simulink model "TotalAssemblyV4"  (R2020b)
settings: Solver=VariableStepAuto  StartTime=0.0  StopTime=10.0  RelTol=1e-3
model workspace: external: MATLAB File C:\Users\User\Aalborg Universitet\ROB 3 - General\P3\Solidworks_files\SimScapeV4\TotalAssemblyV4_DataFile.m (data not in the file)
undefined symbols (not defined in the file or in its folder): smiData, X, Y, Z
libraries: sm_lib x112, simulink_extras x16, nesl_utility x13
(part 3 of 3)

== system TotalAssemblyV4/Body3_3_RIGID/Servo_Disc_3_RIGID ==
  ReferenceFrame : sm_lib/Frames and Transforms/Reference Frame
  Solid : sm_lib/Body Elements/File Solid  ExtGeomFileName=Servo-Disc_Default_sldprt.STEP  UnitType=FromFile  ExtGeomFileUnits=m  StepReaderType=HEX  ExportConvexHullGeometry=off  InertiaType=Custom  Mass=smiData.Solid(2).mass  MassUnits=kg  CenterOfMass=smiData.Solid(2).CoM  CenterOfMassUnits=mm  MomentsOfInertia=smiData.Solid(2).MoI  MomentsOfInertiaUnits=kg*mm^2  ProductsOfInertia=smiData.Solid(2).PoI  ProductsOfInertiaUnits=kg*mm^2  BasedOnType=DensityFromFile  Density=1000  DensityUnits=kg/m^3  DoExposeReferenceFrame=on  SerializedFrames=<Frames/>  GraphicType=FromGeometry  MarkerShape=Sphere  MarkerSize=10  GraphicVisPropType=SimpleVisualProperties  GraphicDiffuseColor=smiData.Solid(2).color  GraphicSpecularColor=[0.5 0.5 0.5 1.0]  GraphicAmbientColor=[0.15 0.15 0.15 1.0]  GraphicEmissiveColor=[0.0 0.0 0.0 1.0]  GraphicShininess=75  GraphicOpacity=smiData.Solid(2).opacity
  F : PMIOPort  Side=Left
  connections:
  Solid/RConn1 -- ReferenceFrame/RConn1 -- F/RConn1

== system TotalAssemblyV4/Body3_3_RIGID/Servo_Disc_4_RIGID ==
  ReferenceFrame : sm_lib/Frames and Transforms/Reference Frame
  Solid : sm_lib/Body Elements/File Solid  ExtGeomFileName=Servo-Disc_Default_sldprt.STEP  UnitType=FromFile  ExtGeomFileUnits=m  StepReaderType=HEX  ExportConvexHullGeometry=off  InertiaType=Custom  Mass=smiData.Solid(2).mass  MassUnits=kg  CenterOfMass=smiData.Solid(2).CoM  CenterOfMassUnits=mm  MomentsOfInertia=smiData.Solid(2).MoI  MomentsOfInertiaUnits=kg*mm^2  ProductsOfInertia=smiData.Solid(2).PoI  ProductsOfInertiaUnits=kg*mm^2  BasedOnType=DensityFromFile  Density=1000  DensityUnits=kg/m^3  DoExposeReferenceFrame=on  SerializedFrames=<Frames/>  GraphicType=FromGeometry  MarkerShape=Sphere  MarkerSize=10  GraphicVisPropType=SimpleVisualProperties  GraphicDiffuseColor=smiData.Solid(2).color  GraphicSpecularColor=[0.5 0.5 0.5 1.0]  GraphicAmbientColor=[0.15 0.15 0.15 1.0]  GraphicEmissiveColor=[0.0 0.0 0.0 1.0]  GraphicShininess=75  GraphicOpacity=smiData.Solid(2).opacity
  F : PMIOPort  Side=Left
  connections:
  Solid/RConn1 -- ReferenceFrame/RConn1 -- F/RConn1

== system TotalAssemblyV4/Body3_3_RIGID/Servo_Disc_5_RIGID ==
  ReferenceFrame : sm_lib/Frames and Transforms/Reference Frame
  Solid : sm_lib/Body Elements/File Solid  ExtGeomFileName=Servo-Disc_Default_sldprt.STEP  UnitType=FromFile  ExtGeomFileUnits=m  StepReaderType=HEX  ExportConvexHullGeometry=off  InertiaType=Custom  Mass=smiData.Solid(2).mass  MassUnits=kg  CenterOfMass=smiData.Solid(2).CoM  CenterOfMassUnits=mm  MomentsOfInertia=smiData.Solid(2).MoI  MomentsOfInertiaUnits=kg*mm^2  ProductsOfInertia=smiData.Solid(2).PoI  ProductsOfInertiaUnits=kg*mm^2  BasedOnType=DensityFromFile  Density=1000  DensityUnits=kg/m^3  DoExposeReferenceFrame=on  SerializedFrames=<Frames/>  GraphicType=FromGeometry  MarkerShape=Sphere  MarkerSize=10  GraphicVisPropType=SimpleVisualProperties  GraphicDiffuseColor=smiData.Solid(2).color  GraphicSpecularColor=[0.5 0.5 0.5 1.0]  GraphicAmbientColor=[0.15 0.15 0.15 1.0]  GraphicEmissiveColor=[0.0 0.0 0.0 1.0]  GraphicShininess=75  GraphicOpacity=smiData.Solid(2).opacity
  F : PMIOPort  Side=Left
  connections:
  Solid/RConn1 -- ReferenceFrame/RConn1 -- F/RConn1

== system TotalAssemblyV4/Body3_3_RIGID/Servo_Disc_6_RIGID ==
  ReferenceFrame : sm_lib/Frames and Transforms/Reference Frame
  Solid : sm_lib/Body Elements/File Solid  ExtGeomFileName=Servo-Disc_Default_sldprt.STEP  UnitType=FromFile  ExtGeomFileUnits=m  StepReaderType=HEX  ExportConvexHullGeometry=off  InertiaType=Custom  Mass=smiData.Solid(2).mass  MassUnits=kg  CenterOfMass=smiData.Solid(2).CoM  CenterOfMassUnits=mm  MomentsOfInertia=smiData.Solid(2).MoI  MomentsOfInertiaUnits=kg*mm^2  ProductsOfInertia=smiData.Solid(2).PoI  ProductsOfInertiaUnits=kg*mm^2  BasedOnType=DensityFromFile  Density=1000  DensityUnits=kg/m^3  DoExposeReferenceFrame=on  SerializedFrames=<Frames/>  GraphicType=FromGeometry  MarkerShape=Sphere  MarkerSize=10  GraphicVisPropType=SimpleVisualProperties  GraphicDiffuseColor=smiData.Solid(2).color  GraphicSpecularColor=[0.5 0.5 0.5 1.0]  GraphicAmbientColor=[0.15 0.15 0.15 1.0]  GraphicEmissiveColor=[0.0 0.0 0.0 1.0]  GraphicShininess=75  GraphicOpacity=smiData.Solid(2).opacity
  F : PMIOPort  Side=Left
  connections:
  Solid/RConn1 -- ReferenceFrame/RConn1 -- F/RConn1

== system TotalAssemblyV4/Body3_3_RIGID/Servo_disc_link_MX_28T_1_RIGID ==
  ReferenceFrame : sm_lib/Frames and Transforms/Reference Frame
  Solid : sm_lib/Body Elements/File Solid  ExtGeomFileName=Servo-disc-link_MX-28T_Default_sldprt.STEP  UnitType=FromFile  ExtGeomFileUnits=m  StepReaderType=HEX  ExportConvexHullGeometry=off  InertiaType=Custom  Mass=smiData.Solid(15).mass  MassUnits=kg  CenterOfMass=smiData.Solid(15).CoM  CenterOfMassUnits=mm  MomentsOfInertia=smiData.Solid(15).MoI  MomentsOfInertiaUnits=kg*mm^2  ProductsOfInertia=smiData.Solid(15).PoI  ProductsOfInertiaUnits=kg*mm^2  BasedOnType=DensityFromFile  Density=1000  DensityUnits=kg/m^3  DoExposeReferenceFrame=on  SerializedFrames=<Frames/>  GraphicType=FromGeometry  MarkerShape=Sphere  MarkerSize=10  GraphicVisPropType=SimpleVisualProperties  GraphicDiffuseColor=smiData.Solid(15).color  GraphicSpecularColor=[0.5 0.5 0.5 1.0]  GraphicAmbientColor=[0.15 0.15 0.15 1.0]  GraphicEmissiveColor=[0.0 0.0 0.0 1.0]  GraphicShininess=75  GraphicOpacity=smiData.Solid(15).opacity
  F : PMIOPort  Side=Left
  connections:
  Solid/RConn1 -- ReferenceFrame/RConn1 -- F/RConn1

== system TotalAssemblyV4/Body3_3_RIGID/Servo_disc_link_MX_28T_2_RIGID ==
  ReferenceFrame : sm_lib/Frames and Transforms/Reference Frame
  Solid : sm_lib/Body Elements/File Solid  ExtGeomFileName=Servo-disc-link_MX-28T_Default_sldprt.STEP  UnitType=FromFile  ExtGeomFileUnits=m  StepReaderType=HEX  ExportConvexHullGeometry=off  InertiaType=Custom  Mass=smiData.Solid(15).mass  MassUnits=kg  CenterOfMass=smiData.Solid(15).CoM  CenterOfMassUnits=mm  MomentsOfInertia=smiData.Solid(15).MoI  MomentsOfInertiaUnits=kg*mm^2  ProductsOfInertia=smiData.Solid(15).PoI  ProductsOfInertiaUnits=kg*mm^2  BasedOnType=DensityFromFile  Density=1000  DensityUnits=kg/m^3  DoExposeReferenceFrame=on  SerializedFrames=<Frames/>  GraphicType=FromGeometry  MarkerShape=Sphere  MarkerSize=10  GraphicVisPropType=SimpleVisualProperties  GraphicDiffuseColor=smiData.Solid(15).color  GraphicSpecularColor=[0.5 0.5 0.5 1.0]  GraphicAmbientColor=[0.15 0.15 0.15 1.0]  GraphicEmissiveColor=[0.0 0.0 0.0 1.0]  GraphicShininess=75  GraphicOpacity=smiData.Solid(15).opacity
  F : PMIOPort  Side=Left
  connections:
  Solid/RConn1 -- ReferenceFrame/RConn1 -- F/RConn1

== system TotalAssemblyV4/Body3_3_RIGID/Servo_disc_link_MX_64T_1_RIGID ==
  ReferenceFrame : sm_lib/Frames and Transforms/Reference Frame
  Solid : sm_lib/Body Elements/File Solid  ExtGeomFileName=Servo-disc-link_MX-64T_Default_sldprt.STEP  UnitType=FromFile  ExtGeomFileUnits=m  StepReaderType=HEX  ExportConvexHullGeometry=off  InertiaType=Custom  Mass=smiData.Solid(12).mass  MassUnits=kg  CenterOfMass=smiData.Solid(12).CoM  CenterOfMassUnits=mm  MomentsOfInertia=smiData.Solid(12).MoI  MomentsOfInertiaUnits=kg*mm^2  ProductsOfInertia=smiData.Solid(12).PoI  ProductsOfInertiaUnits=kg*mm^2  BasedOnType=DensityFromFile  Density=1000  DensityUnits=kg/m^3  DoExposeReferenceFrame=on  SerializedFrames=<Frames/>  GraphicType=FromGeometry  MarkerShape=Sphere  MarkerSize=10  GraphicVisPropType=SimpleVisualProperties  GraphicDiffuseColor=smiData.Solid(12).color  GraphicSpecularColor=[0.5 0.5 0.5 1.0]  GraphicAmbientColor=[0.15 0.15 0.15 1.0]  GraphicEmissiveColor=[0.0 0.0 0.0 1.0]  GraphicShininess=75  GraphicOpacity=smiData.Solid(12).opacity
  F : PMIOPort  Side=Left
  connections:
  Solid/RConn1 -- ReferenceFrame/RConn1 -- F/RConn1

== system TotalAssemblyV4/Body3_3_RIGID/Servo_link_link_MX_28T_4_RIGID ==
  ReferenceFrame : sm_lib/Frames and Transforms/Reference Frame
  Solid : sm_lib/Body Elements/File Solid  ExtGeomFileName=Servo-link-link_MX-28T_Default_sldprt.STEP  UnitType=FromFile  ExtGeomFileUnits=m  StepReaderType=HEX  ExportConvexHullGeometry=off  InertiaType=Custom  Mass=smiData.Solid(14).mass  MassUnits=kg  CenterOfMass=smiData.Solid(14).CoM  CenterOfMassUnits=mm  MomentsOfInertia=smiData.Solid(14).MoI  MomentsOfInertiaUnits=kg*mm^2  ProductsOfInertia=smiData.Solid(14).PoI  ProductsOfInertiaUnits=kg*mm^2  BasedOnType=DensityFromFile  Density=1000  DensityUnits=kg/m^3  DoExposeReferenceFrame=on  SerializedFrames=<Frames/>  GraphicType=FromGeometry  MarkerShape=Sphere  MarkerSize=10  GraphicVisPropType=SimpleVisualProperties  GraphicDiffuseColor=smiData.Solid(14).color  GraphicSpecularColor=[0.5 0.5 0.5 1.0]  GraphicAmbientColor=[0.15 0.15 0.15 1.0]  GraphicEmissiveColor=[0.0 0.0 0.0 1.0]  GraphicShininess=75  GraphicOpacity=smiData.Solid(14).opacity
  F : PMIOPort  Side=Left
  connections:
  Solid/RConn1 -- ReferenceFrame/RConn1 -- F/RConn1

== system TotalAssemblyV4/TableAssembly_2_RIGID/Base_1_RIGID ==
  ReferenceFrame : sm_lib/Frames and Transforms/Reference Frame
  Solid : sm_lib/Body Elements/File Solid  ExtGeomFileName=Base_Default_sldprt.STEP  UnitType=FromFile  ExtGeomFileUnits=m  StepReaderType=HEX  ExportConvexHullGeometry=off  InertiaType=Custom  Mass=smiData.Solid(7).mass  MassUnits=kg  CenterOfMass=smiData.Solid(7).CoM  CenterOfMassUnits=mm  MomentsOfInertia=smiData.Solid(7).MoI  MomentsOfInertiaUnits=kg*mm^2  ProductsOfInertia=smiData.Solid(7).PoI  ProductsOfInertiaUnits=kg*mm^2  BasedOnType=DensityFromFile  Density=1000  DensityUnits=kg/m^3  DoExposeReferenceFrame=on  SerializedFrames=<Frames/>  GraphicType=FromGeometry  MarkerShape=Sphere  MarkerSize=10  GraphicVisPropType=SimpleVisualProperties  GraphicDiffuseColor=smiData.Solid(7).color  GraphicSpecularColor=[0.5 0.5 0.5 1.0]  GraphicAmbientColor=[0.15 0.15 0.15 1.0]  GraphicEmissiveColor=[0.0 0.0 0.0 1.0]  GraphicShininess=75  GraphicOpacity=smiData.Solid(7).opacity
  F : PMIOPort  Side=Left
  connections:
  Solid/RConn1 -- ReferenceFrame/RConn1 -- F/RConn1

== system TotalAssemblyV4/TableAssembly_2_RIGID/MX_64T_1_RIGID ==
  ReferenceFrame : sm_lib/Frames and Transforms/Reference Frame
  Solid : sm_lib/Body Elements/File Solid  ExtGeomFileName=MX-64T_Default_sldprt.STEP  UnitType=FromFile  ExtGeomFileUnits=m  StepReaderType=HEX  ExportConvexHullGeometry=off  InertiaType=Custom  Mass=smiData.Solid(1).mass  MassUnits=kg  CenterOfMass=smiData.Solid(1).CoM  CenterOfMassUnits=mm  MomentsOfInertia=smiData.Solid(1).MoI  MomentsOfInertiaUnits=kg*mm^2  ProductsOfInertia=smiData.Solid(1).PoI  ProductsOfInertiaUnits=kg*mm^2  BasedOnType=DensityFromFile  Density=1000  DensityUnits=kg/m^3  DoExposeReferenceFrame=on  SerializedFrames=<Frames/>  GraphicType=FromGeometry  MarkerShape=Sphere  MarkerSize=10  GraphicVisPropType=SimpleVisualProperties  GraphicDiffuseColor=smiData.Solid(1).color  GraphicSpecularColor=[0.5 0.5 0.5 1.0]  GraphicAmbientColor=[0.15 0.15 0.15 1.0]  GraphicEmissiveColor=[0.0 0.0 0.0 1.0]  GraphicShininess=75  GraphicOpacity=smiData.Solid(1).opacity
  F : PMIOPort  Side=Left
  connections:
  Solid/RConn1 -- ReferenceFrame/RConn1 -- F/RConn1

== matlab function TotalAssemblyV4/Subsystem3/MATLAB Function6 ==
  data: x output; theta1 input; y output; theta2 input; theta3 input; z output
function [x, y, z]= ForwardKinematics(theta1, theta2, theta3)

%TDH(alpha,a,d,theta)


DH = [       0,         0,               0.0528,                theta1;
             -pi/2,    0,                   0,                   theta2;
             0,    0.21988,                   0,                theta3];
%%Transformation matrix from frame 6 to Wrist    
T3_W=[  1,  0,  0,  0.22368;
        0,  1, 0,  0;
        0,  0,  1, 0;
        0,  0,  0,  1];
    
outputMatrice = DH_toMatrice(DH,1,3)*T3_W; %Returns transformation matrix from specified Joint to wrist

x = outputMatrice(1,4);
y = outputMatrice(2,4);
z = outputMatrice(3,4);
end

== matlab function TotalAssemblyV4/MATLAB Function1 ==
  data: theta1a output; x input; theta2a output; y input; z input; theta3a output; theta1b output; theta2b output; theta3b output; theta1c output; theta2c output; theta3c output; theta1d output; theta2d output; theta3d output
function [theta1a, theta2a, theta3a, theta1b, theta2b, theta3b, theta1c, theta2c, theta3c, theta1d, theta2d, theta3d]= InverseKinematics(x, y, z)
    L1 = 0.0528;
    L2 = 0.21988;
    L3 = 0.22368;
    %Thete1 er godkendt med 2 værdier
    theta1a=((atan2(y,x)));
    theta1b=theta1a+pi;
    theta1c = theta1a;
    theta1d = theta1b;
    
    r = sqrt((x^2)+(y^2));
    c = sqrt((z-L1)^2+r^2);
    a=atan2(z-L1,r);
    A=acos((c^2+L2^2-L3^2)/(2*c*L2));
    
    %
    theta2a = -(a+A);
    theta2b = +(a+A)-pi;
    %theta2c = -(a+(2*pi-A))+2*pi;
    theta2c = A-a;
    theta2d = a-A-pi;
    
    theta3 = acos((L3^2+L2^2-c^2)/(2*L3*L2));
    theta3a = pi-theta3;
    theta3b = -pi+theta3;
    theta3c = -pi+theta3;
    theta3d = pi-theta3;
    
    %theta3a = acos((c^2-L3^2-L2^2)/(2*L3*L2));
   % theta3b = acos((c^2-L3^2-L2^2)/(2*L3*L2));
   % T3=rad2deg(theta3a);
    
   % theta2a = atan2(r, z-L1)-atan2(L2+L3*cos(theta3a), L3*sin(theta3a));
   % theta2b = atan2(r, z-L1)+atan2(L2+L3*cos(theta3b), L3*sin(theta3b));
 
     
        
    T2=rad2deg(theta2a);
    
end

== matlab function TotalAssemblyV4/MATLAB Function ==
  data: x output; theta1 input; y output; theta2 input; theta3 input; z output
function [x, y, z]= ForwardKinematics(theta1, theta2, theta3)

%TDH(alpha,a,d,theta)


DH = [       0,         0,               0.0528,                theta1;
             -pi/2,    0,                   0,                   theta2;
             0,    0.21988,                   0,                theta3];
%%Transformation matrix from frame 6 to Wrist    
T3_W=[  1,  0,  0,  0.22368;
        0,  1, 0,  0;
        0,  0,  1, 0;
        0,  0,  0,  1];
    
outputMatrice = DH_toMatrice(DH,1,3)*T3_W; %Returns transformation matrix from specified Joint to wrist

x = outputMatrice(1,4);
y = outputMatrice(2,4);
z = outputMatrice(3,4);
end

== matlab function TotalAssemblyV4/MATLAB Function2 ==
  data: tau1 output; theta1 input; tau2 output; theta2 input; theta3 input; tau3 output; dtheta1 input; dtheta2 input; dtheta3 input; ddtheta1 input; ddtheta2 input; ddtheta3 input
function [tau1, tau2, tau3]=Inversedynamaics(theta1, theta2, theta3, dtheta1, dtheta2, dtheta3, ddtheta1, ddtheta2, ddtheta3)

tau1 = 0.020477058988725499418764229305867*ddtheta1 - 0.0088297863675*ddtheta1*cos(2.0*theta2 + theta3) + 0.000045525453907039896436459509889104*dtheta2^2*sin(2.0*theta2 - 0.069813170079773183076947630739545*theta1) - 0.000045525453907039896436459509889104*dtheta2^2*sin(0.069813170079773183076947630739545*theta1 + 2.0*theta2) + 0.00001225666622146713894713577797915*dtheta2^2*sin(2.0*theta2 - 0.069813170079773183076947630739545*theta1 + 2.0*theta3) - 0.00001225666622146713894713577797915*dtheta2^2*sin(0.069813170079773183076947630739545*theta1 + 2.0*theta2 + 2.0*theta3) + 0.00001225666622146713894713577797915*dtheta3^2*sin(2.0*theta2 - 0.069813170079773183076947630739545*theta1 + 2.0*theta3) - 0.00001225666622146713894713577797915*dtheta3^2*sin(0.069813170079773183076947630739545*theta1 + 2.0*theta2 + 2.0*theta3) - 0.0066126016171630002306207632502*ddtheta1*cos(2.0*theta2) - 0.000011588219999999999987663756861878*ddtheta1*sin(2.0*theta2) + 0.000000047789999999999999785588042843995*ddtheta2*cos(theta2 + theta3) + 0.000000047789999999999999785588042843995*ddtheta3*cos(theta2 + theta3) - 0.000032669149999999998743634849196482*ddtheta2*sin(theta2 + theta3) - 0.000032669149999999998743634849196482*ddtheta3*sin(theta2 + theta3) + 0.000038527211090146258714057118338466*dtheta2^2*sin(theta3 - 0.069813170079773183076947630739545*theta1) - 0.000038527211090146258714057118338466*dtheta2^2*sin(0.069813170079773183076947630739545*theta1 + theta3) + 0.000038527211090146258714057118338466*dtheta2^2*sin(2.0*theta2 - 0.069813170079773183076947630739545*theta1 + theta3) - 0.000038527211090146258714057118338466*dtheta2^2*sin(0.069813170079773183076947630739545*theta1 + 2.0*theta2 + theta3) + 0.0088297863675*ddtheta1*cos(theta3) - 0.000017807919999999997375493554496728*ddtheta2*sin(theta2) + 0.00028211581843749966055163752587376*ddtheta1*cos(2.0*theta2 + 2.0*theta3) - 0.00011556424025701407076719057573651*dtheta2^2*sin(0.069813170079773183076947630739545*theta1) - 0.000024513332442934277894271555958301*dtheta3^2*sin(0.069813170079773183076947630739545*theta1) + 0.000000071470000000000004039742986742395*ddtheta1*sin(2.0*theta2 + 2.0*theta3) - 0.000032669149999999998743634849196482*dtheta2^2*cos(theta2 + theta3) - 0.000032669149999999998743634849196482*dtheta3^2*cos(theta2 + theta3) - 0.000000047789999999999999785588042843995*dtheta2^2*sin(theta2 + theta3) - 0.000000047789999999999999785588042843995*dtheta3^2*sin(theta2 + theta3) - 0.000017807919999999997375493554496728*dtheta2^2*cos(theta2) - 0.0088297863675*dtheta1*dtheta3*sin(theta3) + 0.00000014294000000000000807948597348479*dtheta1*dtheta2*cos(2.0*theta2 + 2.0*theta3) + 0.00000014294000000000000807948597348479*dtheta1*dtheta3*cos(2.0*theta2 + 2.0*theta3) - 0.00056423163687499932110327505174752*dtheta1*dtheta2*sin(2.0*theta2 + 2.0*theta3) - 0.00056423163687499932110327505174752*dtheta1*dtheta3*sin(2.0*theta2 + 2.0*theta3) + 0.000024513332442934277894271555958301*dtheta2*dtheta3*sin(2.0*theta2 - 0.069813170079773183076947630739545*theta1 + 2.0*theta3) - 0.000024513332442934277894271555958301*dtheta2*dtheta3*sin(0.069813170079773183076947630739545*theta1 + 2.0*theta2 + 2.0*theta3) + 0.017659572735*dtheta1*dtheta2*sin(2.0*theta2 + theta3) + 0.0088297863675*dtheta1*dtheta3*sin(2.0*theta2 + theta3) + 0.000038527211090146258714057118338466*dtheta2*dtheta3*sin(theta3 - 0.069813170079773183076947630739545*theta1) - 0.000038527211090146258714057118338466*dtheta2*dtheta3*sin(0.069813170079773183076947630739545*theta1 + theta3) + 0.000038527211090146258714057118338466*dtheta2*dtheta3*sin(2.0*theta2 - 0.069813170079773183076947630739545*theta1 + theta3) - 0.000038527211090146258714057118338466*dtheta2*dtheta3*sin(0.069813170079773183076947630739545*theta1 + 2.0*theta2 + theta3) - 0.000023176439999999999975327513723755*dtheta1*dtheta2*cos(2.0*theta2) + 0.0132252032343260004612415265004*dtheta1*dtheta2*sin(2.0*theta2) - 0.000049026664885868555788543111916601*dtheta2*dtheta3*sin(0.069813170079773183076947630739545*theta1) - 0.000065338299999999997487269698392964*dtheta2*dtheta3*cos(theta2 + theta3) - 0.00000009557999999999999957117608568799*dtheta2*dtheta3*sin(theta2 + theta3)


 
tau2 = 0.017238061144681375572584895053296*ddtheta2 + 0.0069535131453906253878745324925603*ddtheta3 - 0.99879132209199995871440336259184*cos(theta2) - 0.0011037232959375*dtheta3^2*sin(theta3) - 0.39448818074999999179208742816627*cos(theta2)*cos(theta3) + 0.39448818074999999179208742816627*sin(theta2)*sin(theta3) + 0.00260841636929075*ddtheta2*cos(2.0*theta2) - 0.003310671614681375*ddtheta2*cos(0.069813170079773183076947630739545*theta1) - 0.000702255245390625*ddtheta3*cos(0.069813170079773183076947630739545*theta1) + 0.000011588219999999999987663756861878*dtheta1^2*cos(2.0*theta2) + 0.002207446591875*ddtheta2*cos(theta3) + 0.0011037232959375*ddtheta3*cos(theta3) - 0.0066126016171630002306207632502*dtheta1^2*sin(2.0*theta2) - 0.00260841636929075*dtheta2^2*sin(2.0*theta2) - 0.000017807919999999997375493554496728*ddtheta1*sin(theta2) - 0.002207446591875*dtheta2*dtheta3*sin(theta3) - 0.000000071470000000000004039742986742395*dtheta1^2*cos(2.0*theta2)*cos(2.0*theta3) + 0.002207446591875*ddtheta2*cos(2.0*theta2)*cos(theta3) + 0.0011037232959375*ddtheta3*cos(2.0*theta2)*cos(theta3) - 0.002207446591875*ddtheta2*cos(0.069813170079773183076947630739545*theta1)*cos(theta3) - 0.0011037232959375*ddtheta3*cos(0.069813170079773183076947630739545*theta1)*cos(theta3) + 0.00028211581843749966055163752587376*dtheta1^2*cos(2.0*theta2)*sin(2.0*theta3) + 0.00028211581843749966055163752587376*dtheta1^2*cos(2.0*theta3)*sin(2.0*theta2) - 0.000702255245390625*dtheta2^2*cos(2.0*theta2)*sin(2.0*theta3) - 0.000702255245390625*dtheta2^2*cos(2.0*theta3)*sin(2.0*theta2) - 0.000702255245390625*dtheta3^2*cos(2.0*theta2)*sin(2.0*theta3) - 0.000702255245390625*dtheta3^2*cos(2.0*theta3)*sin(2.0*theta2) + 0.00260841636929075*dtheta2^2*cos(0.069813170079773183076947630739545*theta1)*sin(2.0*theta2) + 0.000000071470000000000004039742986742395*dtheta1^2*sin(2.0*theta2)*sin(2.0*theta3) - 0.002207446591875*ddtheta2*sin(2.0*theta2)*sin(theta3) - 0.0011037232959375*ddtheta3*sin(2.0*theta2)*sin(theta3) + 0.000000047789999999999999785588042843995*ddtheta1*cos(theta2)*cos(theta3) - 0.0088297863675*dtheta1^2*cos(2.0*theta2)*sin(theta3) - 0.0088297863675*dtheta1^2*sin(2.0*theta2)*cos(theta3) - 0.002207446591875*dtheta2^2*cos(2.0*theta2)*sin(theta3) - 0.002207446591875*dtheta2^2*sin(2.0*theta2)*cos(theta3) - 0.0011037232959375*dtheta3^2*cos(2.0*theta2)*sin(theta3) - 0.0011037232959375*dtheta3^2*sin(2.0*theta2)*cos(theta3) - 0.000032669149999999998743634849196482*ddtheta1*cos(theta2)*sin(theta3) - 0.000032669149999999998743634849196482*ddtheta1*cos(theta3)*sin(theta2) + 0.0011037232959375*dtheta3^2*cos(0.069813170079773183076947630739545*theta1)*sin(theta3) - 0.000000047789999999999999785588042843995*ddtheta1*sin(theta2)*sin(theta3) + 0.000702255245390625*ddtheta2*cos(2.0*theta2)*cos(2.0*theta3) + 0.000702255245390625*ddtheta3*cos(2.0*theta2)*cos(2.0*theta3) + 0.00023112848051402814153438115147302*dtheta1*dtheta2*sin(0.069813170079773183076947630739545*theta1) + 0.000049026664885868555788543111916601*dtheta1*dtheta3*sin(0.069813170079773183076947630739545*theta1) - 0.00260841636929075*ddtheta2*cos(2.0*theta2)*cos(0.069813170079773183076947630739545*theta1) - 0.000702255245390625*ddtheta2*sin(2.0*theta2)*sin(2.0*theta3) - 0.000702255245390625*ddtheta3*sin(2.0*theta2)*sin(2.0*theta3) + 0.002207446591875*dtheta2^2*cos(2.0*theta2)*cos(0.069813170079773183076947630739545*theta1)*sin(theta3) + 0.002207446591875*dtheta2^2*cos(0.069813170079773183076947630739545*theta1)*sin(2.0*theta2)*cos(theta3) + 0.0011037232959375*dtheta3^2*cos(2.0*theta2)*cos(0.069813170079773183076947630739545*theta1)*sin(theta3) + 0.0011037232959375*dtheta3^2*cos(0.069813170079773183076947630739545*theta1)*sin(2.0*theta2)*cos(theta3) - 0.00140451049078125*dtheta2*dtheta3*cos(2.0*theta2)*sin(2.0*theta3) - 0.00140451049078125*dtheta2*dtheta3*cos(2.0*theta3)*sin(2.0*theta2) + 0.00018210181562815958574583803955642*dtheta1*dtheta2*cos(2.0*theta2)*sin(0.069813170079773183076947630739545*theta1) - 0.000702255245390625*ddtheta2*cos(2.0*theta2)*cos(2.0*theta3)*cos(0.069813170079773183076947630739545*theta1) - 0.000702255245390625*ddtheta3*cos(2.0*theta2)*cos(2.0*theta3)*cos(0.069813170079773183076947630739545*theta1) + 0.000702255245390625*ddtheta2*cos(0.069813170079773183076947630739545*theta1)*sin(2.0*theta2)*sin(2.0*theta3) + 0.000702255245390625*ddtheta3*cos(0.069813170079773183076947630739545*theta1)*sin(2.0*theta2)*sin(2.0*theta3) - 0.002207446591875*dtheta2*dtheta3*cos(2.0*theta2)*sin(theta3) - 0.002207446591875*dtheta2*dtheta3*sin(2.0*theta2)*cos(theta3) + 0.00015410884436058503485622847335386*dtheta1*dtheta2*sin(0.069813170079773183076947630739545*theta1)*cos(theta3) + 0.000077054422180292517428114236676932*dtheta1*dtheta3*sin(0.069813170079773183076947630739545*theta1)*cos(theta3) + 0.002207446591875*dtheta2*dtheta3*cos(0.069813170079773183076947630739545*theta1)*sin(theta3) - 0.002207446591875*ddtheta2*cos(2.0*theta2)*cos(0.069813170079773183076947630739545*theta1)*cos(theta3) - 0.0011037232959375*ddtheta3*cos(2.0*theta2)*cos(0.069813170079773183076947630739545*theta1)*cos(theta3) + 0.000702255245390625*dtheta2^2*cos(2.0*theta2)*cos(0.069813170079773183076947630739545*theta1)*sin(2.0*theta3) + 0.000702255245390625*dtheta2^2*cos(2.0*theta3)*cos(0.069813170079773183076947630739545*theta1)*sin(2.0*theta2) + 0.000702255245390625*dtheta3^2*cos(2.0*theta2)*cos(0.069813170079773183076947630739545*theta1)*sin(2.0*theta3) + 0.000702255245390625*dtheta3^2*cos(2.0*theta3)*cos(0.069813170079773183076947630739545*theta1)*sin(2.0*theta2) + 0.002207446591875*ddtheta2*cos(0.069813170079773183076947630739545*theta1)*sin(2.0*theta2)*sin(theta3) + 0.0011037232959375*ddtheta3*cos(0.069813170079773183076947630739545*theta1)*sin(2.0*theta2)*sin(theta3) + 0.00015410884436058503485622847335386*dtheta1*dtheta2*cos(2.0*theta2)*sin(0.069813170079773183076947630739545*theta1)*cos(theta3) + 0.000077054422180292517428114236676932*dtheta1*dtheta3*cos(2.0*theta2)*sin(0.069813170079773183076947630739545*theta1)*cos(theta3) + 0.002207446591875*dtheta2*dtheta3*cos(2.0*theta2)*cos(0.069813170079773183076947630739545*theta1)*sin(theta3) + 0.002207446591875*dtheta2*dtheta3*cos(0.069813170079773183076947630739545*theta1)*sin(2.0*theta2)*cos(theta3) - 0.00015410884436058503485622847335386*dtheta1*dtheta2*sin(2.0*theta2)*sin(0.069813170079773183076947630739545*theta1)*sin(theta3) - 0.000077054422180292517428114236676932*dtheta1*dtheta3*sin(2.0*theta2)*sin(0.069813170079773183076947630739545*theta1)*sin(theta3) + 0.000049026664885868555788543111916601*dtheta1*dtheta2*cos(2.0*theta2)*cos(2.0*theta3)*sin(0.069813170079773183076947630739545*theta1) + 0.000049026664885868555788543111916601*dtheta1*dtheta3*cos(2.0*theta2)*cos(2.0*theta3)*sin(0.069813170079773183076947630739545*theta1) + 0.00140451049078125*dtheta2*dtheta3*cos(2.0*theta2)*cos(0.069813170079773183076947630739545*theta1)*sin(2.0*theta3) + 0.00140451049078125*dtheta2*dtheta3*cos(2.0*theta3)*cos(0.069813170079773183076947630739545*theta1)*sin(2.0*theta2) - 0.000049026664885868555788543111916601*dtheta1*dtheta2*sin(2.0*theta2)*sin(2.0*theta3)*sin(0.069813170079773183076947630739545*theta1) - 0.000049026664885868555788543111916601*dtheta1*dtheta3*sin(2.0*theta2)*sin(2.0*theta3)*sin(0.069813170079773183076947630739545*theta1)


tau3 = 0.0069535131453906253878745324925603*ddtheta2 + 0.0069535131453906253878745324925603*ddtheta3 - 0.39448818074999999179208742816627*cos(theta2 + theta3) + 0.00441489318375*dtheta1^2*sin(theta3) + 0.0011037232959375*dtheta2^2*sin(theta3) - 0.000000071470000000000004039742986742395*dtheta1^2*cos(2.0*theta2 + 2.0*theta3) + 0.0011037232959375*ddtheta2*cos(2.0*theta2 + theta3) - 0.00055186164796875*ddtheta2*cos(theta3 - 0.069813170079773183076947630739545*theta1) - 0.00055186164796875*ddtheta2*cos(0.069813170079773183076947630739545*theta1 + theta3) + 0.00028211581843749966055163752587376*dtheta1^2*sin(2.0*theta2 + 2.0*theta3) - 0.000702255245390625*dtheta2^2*sin(2.0*theta2 + 2.0*theta3) - 0.000702255245390625*dtheta3^2*sin(2.0*theta2 + 2.0*theta3) - 0.00055186164796875*ddtheta2*cos(2.0*theta2 - 0.069813170079773183076947630739545*theta1 + theta3) - 0.00055186164796875*ddtheta2*cos(0.069813170079773183076947630739545*theta1 + 2.0*theta2 + theta3) + 0.0003511276226953125*dtheta2^2*sin(2.0*theta2 - 0.069813170079773183076947630739545*theta1 + 2.0*theta3) + 0.0003511276226953125*dtheta2^2*sin(0.069813170079773183076947630739545*theta1 + 2.0*theta2 + 2.0*theta3) + 0.0003511276226953125*dtheta3^2*sin(2.0*theta2 - 0.069813170079773183076947630739545*theta1 + 2.0*theta3) + 0.0003511276226953125*dtheta3^2*sin(0.069813170079773183076947630739545*theta1 + 2.0*theta2 + 2.0*theta3) - 0.000702255245390625*ddtheta2*cos(0.069813170079773183076947630739545*theta1) - 0.000702255245390625*ddtheta3*cos(0.069813170079773183076947630739545*theta1) + 0.000000047789999999999999785588042843995*ddtheta1*cos(theta2 + theta3) - 0.00441489318375*dtheta1^2*sin(2.0*theta2 + theta3) - 0.0011037232959375*dtheta2^2*sin(2.0*theta2 + theta3) - 0.000032669149999999998743634849196482*ddtheta1*sin(theta2 + theta3) - 0.00055186164796875*dtheta2^2*sin(theta3 - 0.069813170079773183076947630739545*theta1) - 0.00055186164796875*dtheta2^2*sin(0.069813170079773183076947630739545*theta1 + theta3) + 0.00055186164796875*dtheta2^2*sin(2.0*theta2 - 0.069813170079773183076947630739545*theta1 + theta3) + 0.00055186164796875*dtheta2^2*sin(0.069813170079773183076947630739545*theta1 + 2.0*theta2 + theta3) + 0.0011037232959375*ddtheta2*cos(theta3) + 0.000702255245390625*ddtheta2*cos(2.0*theta2 + 2.0*theta3) + 0.000702255245390625*ddtheta3*cos(2.0*theta2 + 2.0*theta3) - 0.0003511276226953125*ddtheta2*cos(2.0*theta2 - 0.069813170079773183076947630739545*theta1 + 2.0*theta3) - 0.0003511276226953125*ddtheta2*cos(0.069813170079773183076947630739545*theta1 + 2.0*theta2 + 2.0*theta3) - 0.0003511276226953125*ddtheta3*cos(2.0*theta2 - 0.069813170079773183076947630739545*theta1 + 2.0*theta3) - 0.0003511276226953125*ddtheta3*cos(0.069813170079773183076947630739545*theta1 + 2.0*theta2 + 2.0*theta3) - 0.00140451049078125*dtheta2*dtheta3*sin(2.0*theta2 + 2.0*theta3) - 0.000024513332442934277894271555958301*dtheta1*dtheta2*sin(2.0*theta2 - 0.069813170079773183076947630739545*theta1 + 2.0*theta3) + 0.000024513332442934277894271555958301*dtheta1*dtheta2*sin(0.069813170079773183076947630739545*theta1 + 2.0*theta2 + 2.0*theta3) - 0.000024513332442934277894271555958301*dtheta1*dtheta3*sin(2.0*theta2 - 0.069813170079773183076947630739545*theta1 + 2.0*theta3) + 0.000024513332442934277894271555958301*dtheta1*dtheta3*sin(0.069813170079773183076947630739545*theta1 + 2.0*theta2 + 2.0*theta3) + 0.000702255245390625*dtheta2*dtheta3*sin(2.0*theta2 - 0.069813170079773183076947630739545*theta1 + 2.0*theta3) + 0.000702255245390625*dtheta2*dtheta3*sin(0.069813170079773183076947630739545*theta1 + 2.0*theta2 + 2.0*theta3) - 0.000038527211090146258714057118338466*dtheta1*dtheta2*sin(theta3 - 0.069813170079773183076947630739545*theta1) + 0.000038527211090146258714057118338466*dtheta1*dtheta2*sin(0.069813170079773183076947630739545*theta1 + theta3) - 0.000038527211090146258714057118338466*dtheta1*dtheta2*sin(2.0*theta2 - 0.069813170079773183076947630739545*theta1 + theta3) + 0.000038527211090146258714057118338466*dtheta1*dtheta2*sin(0.069813170079773183076947630739545*theta1 + 2.0*theta2 + theta3) + 0.000049026664885868555788543111916601*dtheta1*dtheta2*sin(0.069813170079773183076947630739545*theta1) + 0.000049026664885868555788543111916601*dtheta1*dtheta3*sin(0.069813170079773183076947630739545*theta1)



end

== matlab function TotalAssemblyV4/Subsystem/MATLAB Function3 ==
  data: x output; theta1 input; y output; theta2 input; theta3 input; z output
function [x, y, z]= ForwardKinematics(theta1, theta2, theta3)

%TDH(alpha,a,d,theta)


DH = [       0,         0,               0.0528,                theta1;
             -pi/2,    0,                   0,                   theta2;
             0,    0.21988,                   0,                theta3];
%%Transformation matrix from frame 6 to Wrist    
T3_W=[  1,  0,  0,  0.22368;
        0,  1, 0,  0;
        0,  0,  1, 0;
        0,  0,  0,  1];
    
outputMatrice = DH_toMatrice(DH,1,3)*T3_W; %Returns transformation matrix from specified Joint to wrist

x = outputMatrice(1,4);
y = outputMatrice(2,4);
z = outputMatrice(3,4);
end

== matlab function TotalAssemblyV4/Subsystem1/MATLAB Function4 ==
  data: x output; theta1 input; y output; theta2 input; theta3 input; z output
function [x, y, z]= ForwardKinematics(theta1, theta2, theta3)

%TDH(alpha,a,d,theta)


DH = [       0,         0,               0.0528,                theta1;
             -pi/2,    0,                   0,                   theta2;
             0,    0.21988,                   0,                theta3];
%%Transformation matrix from frame 6 to Wrist    
T3_W=[  1,  0,  0,  0.22368;
        0,  1, 0,  0;
        0,  0,  1, 0;
        0,  0,  0,  1];
    
outputMatrice = DH_toMatrice(DH,1,3)*T3_W; %Returns transformation matrix from specified Joint to wrist

x = outputMatrice(1,4);
y = outputMatrice(2,4);
z = outputMatrice(3,4);
end

== matlab function TotalAssemblyV4/Subsystem2/MATLAB Function5 ==
  data: x output; theta1 input; y output; theta2 input; theta3 input; z output
function [x, y, z]= ForwardKinematics(theta1, theta2, theta3)

%TDH(alpha,a,d,theta)


DH = [       0,         0,               0.0528,                theta1;
             -pi/2,    0,                   0,                   theta2;
             0,    0.21988,                   0,                theta3];
%%Transformation matrix from frame 6 to Wrist    
T3_W=[  1,  0,  0,  0.22368;
        0,  1, 0,  0;
        0,  0,  1, 0;
        0,  0,  0,  1];
    
outputMatrice = DH_toMatrice(DH,1,3)*T3_W; %Returns transformation matrix from specified Joint to wrist

x = outputMatrice(1,4);
y = outputMatrice(2,4);
z = outputMatrice(3,4);
end
